simulink model "modelLin"  (R2019b)
settings: Solver=ode45  StartTime=0.0  StopTime=10  MaxStep=0.00001  RelTol=1e-8
undefined symbols (not defined in the file): A, B, C, K
libraries: simulink x1, simulink_extras x1
settings Model: Creator=Mark  LastModifiedBy=Mark

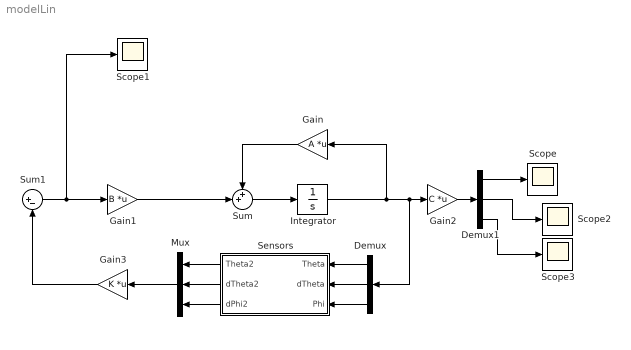
== system modelLin ==
  Demux : Demux  Outputs=3
  Demux1 : Demux  Outputs=3
  Gain : Gain  Gain=A  Multiplication=Matrix(K*u)
  Gain1 : Gain  Gain=B  Multiplication=Matrix(K*u)
  Gain2 : Gain  Gain=C  Multiplication=Matrix(K*u)
  Gain3 : Gain  Gain=K  Multiplication=Matrix(K*u)
  Integrator : Integrator  InitialCondition=[deg2rad(5); 0; 0]
  Mux : Mux  Inputs=3
  Scope{,1..3} (4 alike) : Scope
  Sensors : Subsystem
  Sum : Sum  Inputs=++|
  Sum1 : Sum  Inputs=|+-
  wires:
  Integrator/1 -> Gain2/1, Demux/1, Gain/1
  Gain/1 -> Sum/1
  Gain1/1 -> Sum/2
  Sum/1 -> Integrator/1
  Demux/1 -> Sensors/1(Theta)
  Demux/2 -> Sensors/2(dTheta)
  Demux/3 -> Sensors/3(Phi)
  Mux/1 -> Gain3/1
  Sensors/3(dPhi2) -> Mux/3
  Sensors/1(Theta2) -> Mux/1
  Sensors/2(dTheta2) -> Mux/2
  Sum1/1 -> Scope1/1, Gain1/1
  Gain3/1 -> Sum1/2
  Gain2/1 -> Demux1/1
  Demux1/1 -> Scope/1
  Demux1/2 -> Scope2/1
  Demux1/3 -> Scope3/1

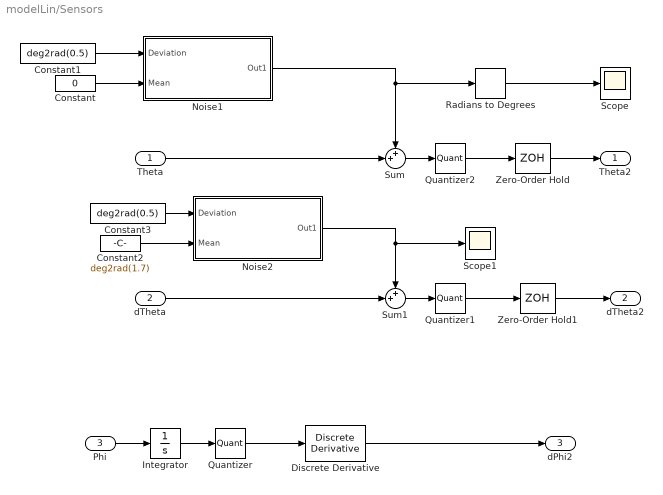
== system modelLin/Sensors ==
  Theta : Inport
  dTheta : Inport  Port=2
  Phi : Inport  Port=3
  Constant : Constant  Value=0
  Constant1 : Constant  Value=deg2rad(0.5)
  Constant2 : Constant  Value=deg2rad(1.7)
  Constant3 : Constant  Value=deg2rad(0.5)
  Discrete Derivative : simulink/Discrete/Discrete Derivative  gainval=1.0  ICPrevScaledInput=0.0  OutMin=[]  OutMax=[]  OutDataType=fixdt(1, 16)  OutScaling=2^-10  DoSatur=off
  Integrator : Integrator
  Noise1 : Subsystem
  Noise2 : Subsystem
  Quantizer : Quantizer  QuantizationInterval=0.00001
  Quantizer1 : Quantizer  QuantizationInterval=0.00001
  Quantizer2 : Quantizer  QuantizationInterval=0.00001
  Radians to Degrees : simulink_extras/Transformations/Radians to Degrees
  Scope : Scope
  Scope1 : Scope
  Sum : Sum  Inputs=++|
  Sum1 : Sum  Inputs=++|
  Zero-Order Hold : ZeroOrderHold  SampleTime=1/1000
  Zero-Order Hold1 : ZeroOrderHold  SampleTime=1/1000
  Theta2 : Outport
  dTheta2 : Outport  Port=2
  dPhi2 : Outport  Port=3
  wires:
  Theta/1 -> Sum/2
  dTheta/1 -> Sum1/2
  Phi/1 -> Integrator/1
  Constant1/1 -> Noise1/1(Deviation)
  Constant/1 -> Noise1/2(Mean)
  Sum/1 -> Quantizer2/1
  Noise1/1(Out1) -> Sum/1, Radians to Degrees/1
  Constant3/1 -> Noise2/1(Deviation)
  Constant2/1 -> Noise2/2(Mean)
  Sum1/1 -> Quantizer1/1
  Noise2/1(Out1) -> Scope1/1, Sum1/1
  Quantizer/1 -> Discrete Derivative/1
  Radians to Degrees/1 -> Scope/1
  Discrete Derivative/1 -> dPhi2/1
  Integrator/1 -> Quantizer/1
  Quantizer2/1 -> Zero-Order Hold/1
  Quantizer1/1 -> Zero-Order Hold1/1
  Zero-Order Hold/1 -> Theta2/1
  Zero-Order Hold1/1 -> dTheta2/1

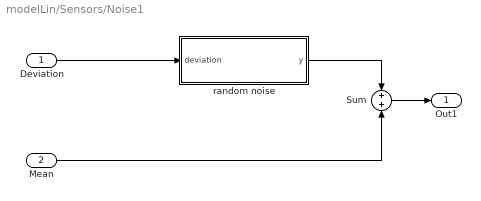
== system modelLin/Sensors/Noise1 ==
  Deviation : Inport
  Mean : Inport  Port=2
  Sum : Sum
  random noise : MATLAB Function  TreatAsAtomicUnit=on  SystemSampleTime=0.001
  Out1 : Outport
  wires:
  Deviation/1 -> random noise/1(deviation)
  random noise/1(y) -> Sum/1
  Mean/1 -> Sum/2
  Sum/1 -> Out1/1

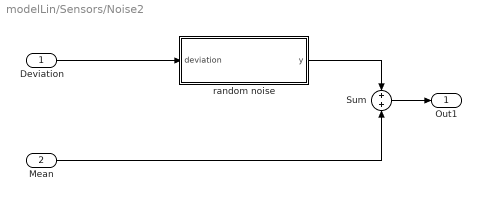
== system modelLin/Sensors/Noise2 ==
  Deviation : Inport
  Mean : Inport  Port=2
  Sum : Sum
  random noise : MATLAB Function  TreatAsAtomicUnit=on  SystemSampleTime=0.001
  Out1 : Outport
  wires:
  Deviation/1 -> random noise/1(deviation)
  random noise/1(y) -> Sum/1
  Mean/1 -> Sum/2
  Sum/1 -> Out1/1

== matlab function modelLin/Sensors/Noise2/random noise ==
  data: y output; deviation input
function y = fcn(deviation)

y = (deviation*randn());

== matlab function modelLin/Sensors/Noise1/random noise ==
  data: y output; deviation input
function y = fcn(deviation)

y = (deviation*randn());
